simulink model "Translational_Dynamics"  (R2018a)
settings: Solver=VariableStepAuto  StartTime=0.0  StopTime=10.0  RelTol=1e-3
libraries: vrlib x1
settings Model: Creator=lamy  LastModifiedBy=lamy

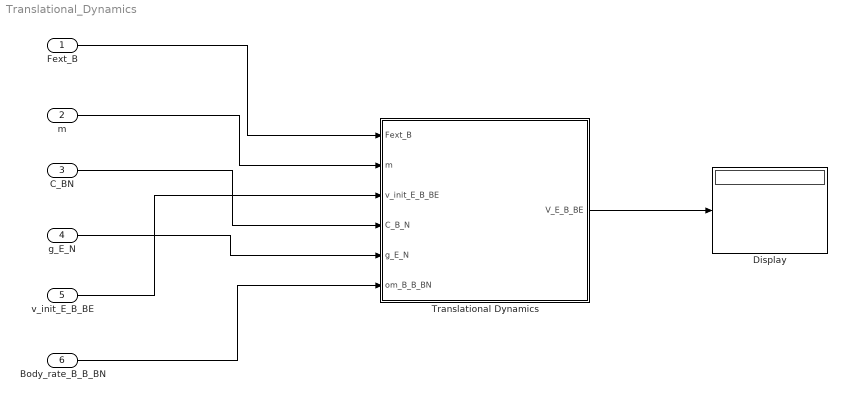
== system Translational_Dynamics ==
  Fext_B : Inport
  m : Inport  Port=2
  C_BN : Inport  Port=3
  g_E_N : Inport  Port=4
  v_init_E_B_BE : Inport  Port=5
  Body_rate_B_B_BN : Inport  Port=6
  Display : Display
  Translational Dynamics : Subsystem
  wires:
  Fext_B/1 -> Translational Dynamics/1(Fext_B)
  m/1 -> Translational Dynamics/2(m)
  v_init_E_B_BE/1 -> Translational Dynamics/3(v_init_E_B_BE)
  C_BN/1 -> Translational Dynamics/4(C_B_N)
  g_E_N/1 -> Translational Dynamics/5(g_E_N)
  Body_rate_B_B_BN/1 -> Translational Dynamics/6(om_B_B_BN)
  Translational Dynamics/1(V_E_B_BE) -> Display/1

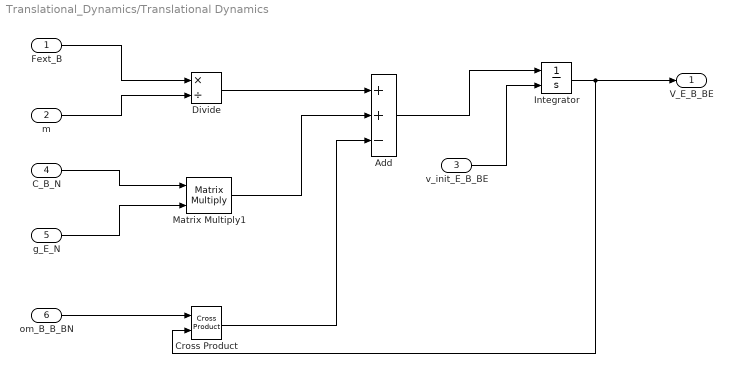
== system Translational_Dynamics/Translational Dynamics ==
  Fext_B : Inport
  m : Inport  Port=2
  v_init_E_B_BE : Inport  Port=3
  C_B_N : Inport  Port=4
  g_E_N : Inport  Port=5
  om_B_B_BN : Inport  Port=6
  Add : Sum  Inputs=++-
  Cross Product : vrlib/Utilities/Cross Product
      settings: SourceProductBaseCode=VR
  Divide : Product  Inputs=*/
  Integrator : Integrator  InitialConditionSource=external
  Matrix Multiply1 : Product  Multiplication=Matrix(*)
  V_E_B_BE : Outport
  wires:
  Cross Product/1 -> Add/3
  Divide/1 -> Add/1
  m/1 -> Divide/2
  Matrix Multiply1/1 -> Add/2
  om_B_B_BN/1 -> Cross Product/1
  Integrator/1 -> V_E_B_BE/1, Cross Product/2
  Fext_B/1 -> Divide/1
  g_E_N/1 -> Matrix Multiply1/2
  v_init_E_B_BE/1 -> Integrator/2
  Add/1 -> Integrator/1
  C_B_N/1 -> Matrix Multiply1/1
